simulink model "m1iv_nonlinearities"  (R2021a)
settings: Solver=VariableStepAuto  StartTime=0.0  StopTime=12  MaxStep=1e-2  RelTol=1e-3
libraries: simulink x8, simulink_extras x8, dspstat3 x2, acolibjan22 x1
settings Model: Creator=jason  LastModifiedBy=jason

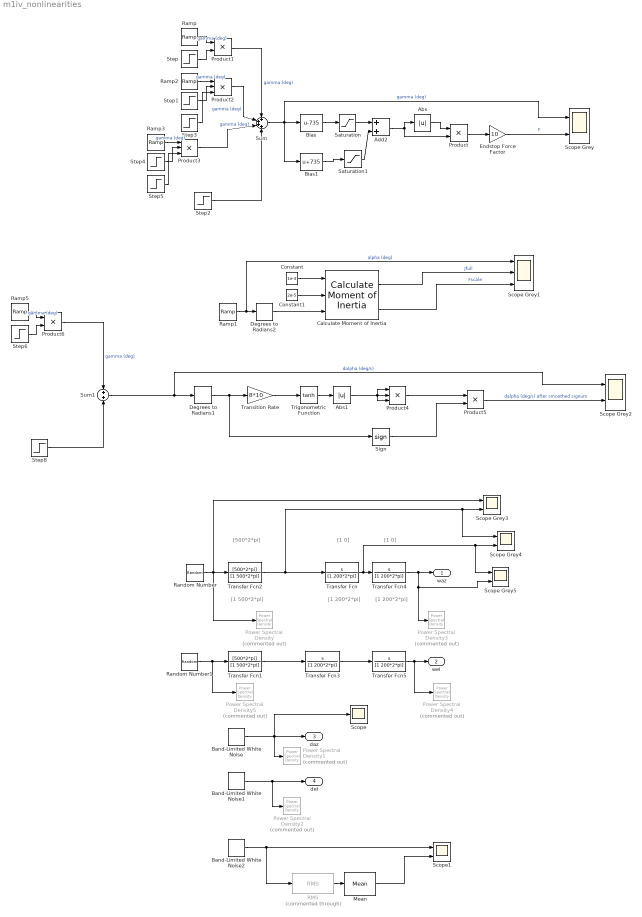
== system m1iv_nonlinearities ==
  note: [1 0]
  note: [1 200*2*pi]
  note: [1 0]
  note: [1 500*2*pi]
  note: [500*2*pi]
  note: [1 200*2*pi]
  Abs : Abs
  Abs1 : Abs
  Add2 : Sum
  Band-Limited White Noise : simulink/Sources/Band-Limited White Noise  Cov=5^2  Ts=0.8  seed=12414
  Band-Limited White Noise1 : simulink/Sources/Band-Limited White Noise  Cov=5^2  Ts=1.2  seed=43214517
  Band-Limited White Noise2 : simulink/Sources/Band-Limited White Noise  Cov=0.1  Ts=0.001  seed=43214517
  Bias : Bias  Bias=-735
  Bias1 : Bias  Bias=735
  Calculate Moment of Inertia : acolibjan22/Plant Model/Sensor Mechanism/Azimuth Equation of Motion/Calculate Moment of Inertia  SystemSampleTime=-1  VariantActivationTime=update diagram  Latency=0  AutoFrameSizeCalculation=off
  Constant : Constant  Value=1e-3
  Constant1 : Constant  Value=2e-5
  Degrees to Radians1 : simulink_extras/Transformations/Degrees to Radians
  Degrees to Radians2 : simulink_extras/Transformations/Degrees to Radians
  Endstop Force Factor : Gain  Gain=10
  Mean : dspstat3/Mean  run=on  InputProcessing=Columns as channels (frame based)  reset_popup=None  directionMode=Entire input  dimension=1  roiEnable=off  roiType=Rectangles  roiPortion=Entire ROI  roiOutput=Individual statistics for each ROI  roiFlag=off  roundingMode=Floor  overflowMode=off  outputDataTypeStr=Inherit: Same as accumulator  outputMin=[]  outputMax=[]  outputLastDataTypeStr=Inherit: Same as accumulator
  Power Spectral Density{,1..5} (6 alike) : simulink_extras/Additional Sinks/Power Spectral Density  Commented=on  npts=128  fftpts=512  HowOften=64  sampleT=0.001
      settings: SourceProductBaseCode=SL
  Product{,1,5..6} (4 alike) : Product
  Product2 : Product  Inputs=3
  Product3 : Product  Inputs=3
  Product4 : Product  Inputs=3
  RMS : dspstat3/RMS  Commented=through  run=off  directionMode=Each column  dimension=1  InputProcessing=Columns as channels (frame based)  reset_popup=None
  Ramp : simulink/Sources/Ramp  slope=1  start=1  InitialOutput=-740
  Ramp1 : simulink/Sources/Ramp  slope=72  start=1  InitialOutput=-360
  Ramp2 : simulink/Sources/Ramp  slope=1  start=6  InitialOutput=735
  Ramp3 : simulink/Sources/Ramp  slope=1470*2  start=5.5  InitialOutput=-735
  Ramp5 : simulink/Sources/Ramp  slope=0.6  start=1  InitialOutput=-3
  Random Number : RandomNumber  Seed=8576  SampleTime=1/1000
  Random Number1 : RandomNumber  Seed=325325  SampleTime=1/500
  Saturation : Saturate  UpperLimit=inf  LowerLimit=0
  Saturation1 : Saturate  UpperLimit=0  LowerLimit=-inf
  Scope : Scope
  Scope Grey{,2..5} (5 alike) : Scope  NumInputPorts=2
  Scope Grey1 : Scope  NumInputPorts=3
  Scope1 : Scope  NumInputPorts=2
  Sign : Signum
  Step : Step  Time=5.5  Before=1  After=0  SampleTime=0
  Step1 : Step  Time=11  Before=1  After=0  SampleTime=0
  Step2 : Step  Time=11  After=740  SampleTime=0
  Step3 : Step  Time=6  SampleTime=0
  Step4 : Step  Time=6  Before=1  After=0  SampleTime=0
  Step5 : Step  Time=5.5  SampleTime=0
  Step6 : Step  Time=11  Before=1  After=0  SampleTime=0
  Step8 : Step  Time=11  After=3  SampleTime=0
  Sum : Sum  Inputs=++++
  Sum1 : Sum  Inputs=+|+
  Transfer Fcn{,3..5} (4 alike) : TransferFcn  Numerator=[1 0]  Denominator=[1 200*2*pi]
  Transfer Fcn1 : TransferFcn  Numerator=[500*2*pi]  Denominator=[1 500*2*pi]
  Transfer Fcn2 : TransferFcn  Numerator=[500*2*pi]  Denominator=[1 500*2*pi]
  Transition Rate : Gain  Gain=8*10
  Trigonometric Function : Trigonometry  Operator=tanh
  waz : Outport  OutputWhenDisabled=reset  InitialOutput=0
  wel : Outport  Port=2  OutputWhenDisabled=reset  InitialOutput=0
  daz : Outport  Port=3  OutputWhenDisabled=reset  InitialOutput=0
  del : Outport  Port=4  OutputWhenDisabled=reset  InitialOutput=0
  wires:
  Bias/1 -> Saturation/1
  Abs/1 -> Product/1
  Add2/1 -> Abs/1, Product/2
  Endstop Force Factor/1 -> Scope Grey/2  "F"
  Sum/1 -> Bias1/1, Scope Grey/1, Bias/1  "gamma (deg)"
  Saturation1/1 -> Add2/2
  Product/1 -> Endstop Force Factor/1
  Saturation/1 -> Add2/1
  Bias1/1 -> Saturation1/1
  Degrees to Radians2/1 -> Calculate Moment of Inertia/3
  Constant1/1 -> Calculate Moment of Inertia/2
  Constant/1 -> Calculate Moment of Inertia/1
  Ramp1/1 -> Scope Grey1/1, Degrees to Radians2/1  "alpha (deg)"
  Calculate Moment of Inertia/2 -> Scope Grey1/3  "Fscale"
  Calculate Moment of Inertia/1 -> Scope Grey1/2  "Jfull"
  Ramp/1 -> Product1/1  "gamma (deg)"
  Step/1 -> Product1/2
  Product1/1 -> Sum/1  "gamma (deg)"
  Step1/1 -> Product2/2
  Ramp2/1 -> Product2/1  "gamma (deg)"
  Product2/1 -> Sum/2  "gamma (deg)"
  Step2/1 -> Sum/4
  Step3/1 -> Product2/3
  Step4/1 -> Product3/2
  Step5/1 -> Product3/3
  Ramp3/1 -> Product3/1  "gamma (deg)"
  Product3/1 -> Sum/3  "gamma (deg)"
  Product5/1 -> Scope Grey2/2  "dalpha (deg/s) after smoothed signum"
  Trigonometric Function/1 -> Abs1/1
  Degrees to Radians1/1 -> Transition Rate/1, Sign/1
  Sign/1 -> Product5/2
  Transition Rate/1 -> Trigonometric Function/1
  Abs1/1 -> Product4/2, Product4/1, Product4/3
  Product4/1 -> Product5/1
  Sum1/1 -> Scope Grey2/1, Degrees to Radians1/1  "dalpha (deg/s)"
  Step6/1 -> Product6/2
  Ramp5/1 -> Product6/1  "gamma (deg)"
  Product6/1 -> Sum1/1  "gamma (deg)"
  Step8/1 -> Sum1/2
  Transfer Fcn4/1 -> Scope Grey5/2, Power Spectral Density3/1, waz/1
  Transfer Fcn/1 -> Scope Grey5/1, Scope Grey4/2, Transfer Fcn4/1
  Transfer Fcn1/1 -> Transfer Fcn3/1
  Transfer Fcn3/1 -> Transfer Fcn5/1
  Transfer Fcn2/1 -> Scope Grey4/1, Scope Grey3/2, Transfer Fcn/1
  Random Number1/1 -> Power Spectral Density5/1, Transfer Fcn1/1
  Random Number/1 -> Power Spectral Density/1, Scope Grey3/1, Transfer Fcn2/1
  Band-Limited White Noise1/1 -> Power Spectral Density2/1, del/1
  Transfer Fcn5/1 -> Power Spectral Density4/1, wel/1
  Band-Limited White Noise/1 -> Scope/1, Power Spectral Density1/1, daz/1
  Band-Limited White Noise2/1 -> RMS/1, Scope1/1
  RMS/1 -> Mean/1
  Mean/1 -> Scope1/2
